simulink model "sim1OscarAvila"  (R2016a)
settings: Solver=ode45  StartTime=0.0  StopTime=Tend  MaxStep=0.01  RelTol=1e-3
values from neighbouring files (symbols this model uses):
  rTs = 0.01    [lab1ControlDigitalOscarAvila.m]
  Ts = 0.005    [dataproyecto.mat]    (also in lab1ControlDigitalOscarAvila.m = 1; practica5.m = 1; proyectoAvilaSilva.m = 3; proyectoAvilaSilva2.m = 3)
  w1 = 1    [lab1ControlDigitalOscarAvila.m]
settings Model: Creator=CltControl  LastModifiedBy=CltControl

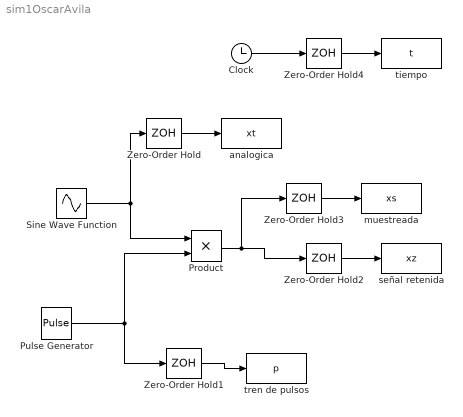
== system sim1OscarAvila ==
  Clock : Clock
  Product : Product
  Pulse Generator : DiscretePulseGenerator  PulseType=Time based  Period=Ts  PulseWidth=0.1
  Sine Wave Function : Sin  Frequency=w1  SampleTime=0
  Zero-Order Hold{,1,3..4} (4 alike) : ZeroOrderHold  SampleTime=rTs
  Zero-Order Hold2 : ZeroOrderHold  SampleTime=Ts
  analogica : ToWorkspace  VariableName=xt  SampleTime=-1
  muestreada : ToWorkspace  VariableName=xs  SampleTime=-1
  señal retenida : ToWorkspace  VariableName=xz  SampleTime=-1
  tiempo : ToWorkspace  VariableName=t  SampleTime=-1
  tren de pulsos : ToWorkspace  VariableName=p  SampleTime=-1
  wires:
  Sine Wave Function/1 -> Product/1, Zero-Order Hold/1
  Pulse Generator/1 -> Zero-Order Hold1/1, Product/2
  Product/1 -> Zero-Order Hold3/1, Zero-Order Hold2/1
  Zero-Order Hold3/1 -> muestreada/1
  Zero-Order Hold2/1 -> señal retenida/1
  Zero-Order Hold1/1 -> tren de pulsos/1
  Clock/1 -> Zero-Order Hold4/1
  Zero-Order Hold4/1 -> tiempo/1
  Zero-Order Hold/1 -> analogica/1
